simulink model "nomoto_model"  (R2017a)
settings: Solver=VariableStepAuto  StartTime=0.0  StopTime=10.0  RelTol=1e-3
undefined symbols (not defined in the file): K, rate_saturation_lower, rate_saturation_upper, saturation_lower, saturation_upper, Tdelta, Tr
settings Model: Creator=Max  LastModifiedBy=Max

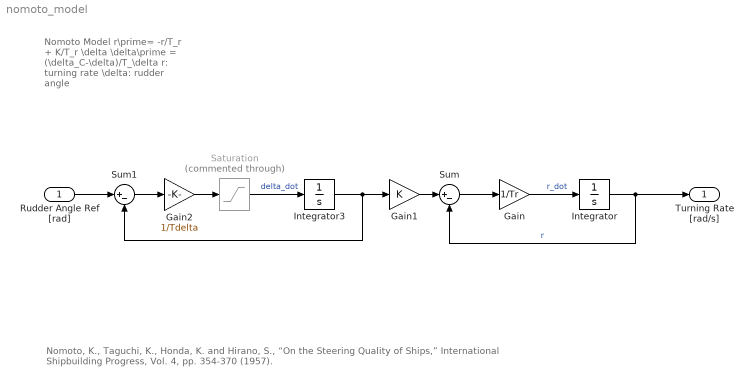
== system nomoto_model ==
  note: Nomoto, K., Taguchi, K., Honda, K. and Hirano, S., “On the Steering Quality of Ships,” International Shipbuilding Progress, Vol. 4, pp. 354-370 (1957).
  note: Nomoto Model
      | r\prime= -r/T_r + K/T_r \delta
      | \delta\prime = (\delta_C-\delta)/T_\delta
      |
      | r: turning rate
      | \delta: rudder angle
  Rudder Angle Ref [rad] : Inport
  Gain : Gain  Gain=1/Tr
  Gain1 : Gain  Gain=K
  Gain2 : Gain  Gain=1/Tdelta
  Integrator : Integrator
  Integrator3 : Integrator  Priority=5  UpperSaturationLimit=saturation_upper  LowerSaturationLimit=saturation_lower  ContinuousStateAttributes='craft_delta'
  Saturation : Saturate  Commented=through  UpperLimit=rate_saturation_upper  LowerLimit=rate_saturation_lower
  Sum : Sum  Inputs=|+-
  Sum1 : Sum  Inputs=|+-
  Turning Rate [rad/s] : Outport
  wires:
  Gain/1 -> Integrator/1  "r_dot"
  Integrator/1 -> Turning Rate [rad/s]/1, Sum/2  "r"
  Gain2/1 -> Saturation/1
  Integrator3/1 -> Sum1/2, Gain1/1
  Sum/1 -> Gain/1
  Gain1/1 -> Sum/1
  Sum1/1 -> Gain2/1
  Rudder Angle Ref [rad]/1 -> Sum1/1
  Saturation/1 -> Integrator3/1  "delta_dot"
